simulink model "PmsmFem_testHarness"  (R2024b)
settings: Solver=daessc  StartTime=0.0  StopTime=0.2  RelTol=1e-3  AbsTol=1e-3
libraries: fl_lib x7, nesl_utility x5, ee_lib x4
settings Model: Creator=The MathWorks, Inc.  LastModifiedBy=isaacito
settings SolverCC: AutoScaleAbsTol=off  AlgebraicLoopSolver=TrustRegion
settings DataIOCC: DSMLogging=off
settings DebuggingCC: UnconnectedInputMsg=warning  UnconnectedOutputMsg=warning  UnconnectedLineMsg=warning  ArithmeticOperatorsInVariantConditions=warning
settings ModelReferenceCC: EnableRefExpFcnMdlSchedulingChecks=on
settings SFSimCC: SimUseLocalCustomCode=off  CustomCodeUndefinedFunction=UseInterfaceOnly
settings RTWCC: RTWUseLocalCustomCode=off  GPUComputeCapability=3.5
settings SimscapeCC: SimscapeLogType=all  SimscapeLogSimulationStatistics=on  SimscapeLogName=logsoutssc  SimscapeLogDataHistory=50000

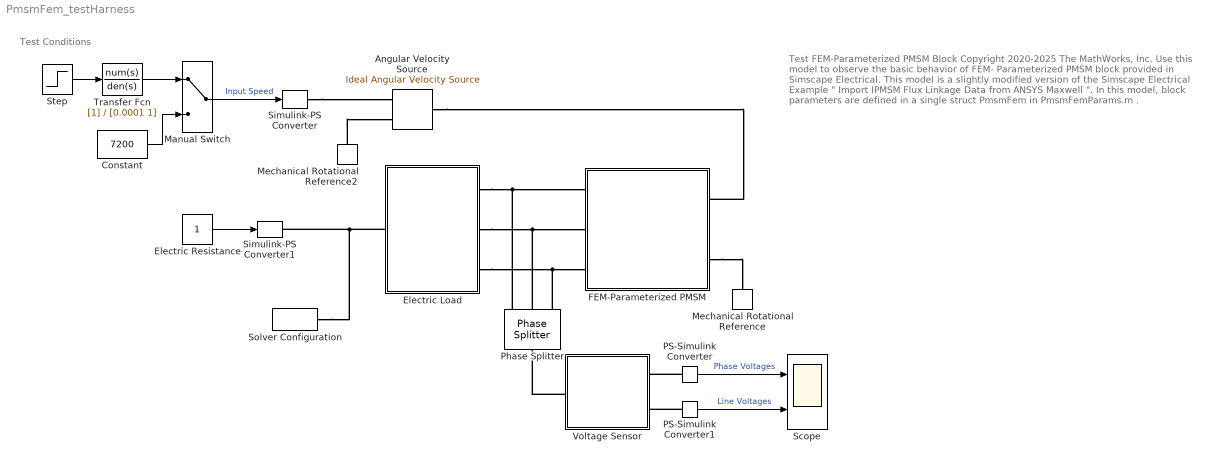
== system PmsmFem_testHarness ==
  note: Test Conditions
  note: Test FEM-Parameterized PMSM Block
      |
      | Copyright 2020-2025 The MathWorks, Inc.
      |
      | Use this model to observe the basic behavior of FEM-
      | Parameterized PMSM block provided in Simscape Electrical.
      | This model is a slightly modified version of the Simscape
      | Electrical Example " Import IPMSM Flux Linkage Data from
      | ANSYS Maxwell ".
      |
      | In this model, block parameters are defined in a single struct
      | PmsmFem in PmsmFemParams.m .
  Angular Velocity Source : fl_lib/Mechanical/Mechanical Sources/Ideal Angular Velocity Source
  Constant : Constant  Value=7200
  Electric Load : Subsystem
  Electric Resistance : Constant
  FEM-Parameterized PMSM : Subsystem  ReferencedSubsystem=PmsmFemRefSub
  Manual Switch : ManualSwitch
  Mechanical Rotational Reference : fl_lib/Mechanical/Rotational Elements/Mechanical Rotational Reference
  Mechanical Rotational Reference2 : fl_lib/Mechanical/Rotational Elements/Mechanical Rotational Reference
  PS-Simulink Converter : nesl_utility/PS-Simulink Converter  PhysicalDomain=network_engine_domain  SubClassName=ps_output  LeftPortType=input  RightPortType=output  PseudoPeriodic=off  Frequencies=[]  VectorFormat=1-D array  Unit=V  AffineConversion=off
  PS-Simulink Converter1 : nesl_utility/PS-Simulink Converter  PhysicalDomain=network_engine_domain  SubClassName=ps_output  LeftPortType=input  RightPortType=output  PseudoPeriodic=off  Frequencies=[]  VectorFormat=1-D array  Unit=V  AffineConversion=off
  Phase Splitter : ee_lib/Connectors & References/Phase Splitter
  Scope : Scope  NumInputPorts=2
  Simulink-PS Converter : nesl_utility/Simulink-PS Converter  PhysicalDomain=network_engine_domain  SubClassName=ps_input  LeftPortType=input  RightPortType=output  PseudoPeriodic=off  Frequencies=[]  NoiseDistribution=none  NoiseParameters=[]  Unit=rpm  AffineConversion=off  FilteringAndDerivatives=filter  SimscapeFilterOrder=1  InputFilterTimeConstant=0.0001  UdotUserProvided=1
  Simulink-PS Converter1 : nesl_utility/Simulink-PS Converter  PhysicalDomain=network_engine_domain  SubClassName=ps_input  LeftPortType=input  RightPortType=output  PseudoPeriodic=off  Frequencies=[]  NoiseDistribution=none  NoiseParameters=[]  Unit=MOhm  AffineConversion=off  FilteringAndDerivatives=provide  SimscapeFilterOrder=1  InputFilterTimeConstant=0.001  UdotUserProvided=0
  Solver Configuration : nesl_utility/Solver Configuration  PhysicalDomain=network_engine_domain  SubClassName=solver  LeftPortType=input  RightPortType=generic  Tones=[]  Harmonics=[]  SimulateNoise=off  Profile=off  UseLocalSampling=off  EnableSwitchedLinearOptims=on  FrequencyDomain=off  UseCCode=off  RelTol=0.001  AbsTol=1e-06  MinStep=1e-09  ToWorkspace=off  RevertToSquareIcSolve=off  NumHomotopyIterations=100  PhasorMode=off  PhasorModeNumHarmonics=1  ConsistencySolver=NEWTON_FTOL  IndexReductionMethod=DerivativeReplacement  DoDC=off  ResidualTolerance=1e-9  ConsistencyTolSource=GLOBAL  ConsistencyAbsTol=0.001  ConsistencyRelTol=0.001  ConsistencyTolFactor=0.001  UseLocalSolver=off  LocalSolverChoice=NE_TRAPEZOIDAL_ADVANCER  ResolveIndetEquations=on  FunctionEvalNumThread=1  LocalSolverSampleTime=0.0001  DoFixedCost=off  MaxNonlinIter=10  MaxModeIter=2  ComputeImpulses=off  ImpulseIterations=2  LinearAlgebra=auto  LinearAlgebraNumThread=0  EquationFormulation=NE_TIME_EF  DelaysMemoryBudget=1024  AutomaticFiltering=on  FilteringTimeConstant=0.001  PartitionStorageMethod=AS_NEEDED  PartitionMemoryBudget=1024  PartitionMethod=FAST  MultibodyUseLocalSolver=off  MultibodyLocalSolverChoice=ODE1  MultibodyLocalSolverSampleTime=0.001
      settings: AttributesFormatString=Local solver %<UseLocalSolver>
  Step : Step  Time=0.1  Before=500  After=1500  SampleTime=0
      settings: AttributesFormatString=|
      | Initial %<Before>
      | Step to %<After>
  Transfer Fcn : TransferFcn  Denominator=[0.0001 1]
  Voltage Sensor : Subsystem
  wires:
  Electric Resistance/1 -> Simulink-PS Converter1/1
  PS-Simulink Converter/1 -> Scope/1  "Phase Voltages"
  PS-Simulink Converter1/1 -> Scope/2  "Line Voltages"
  Manual Switch/1 -> Simulink-PS Converter/1  "Input Speed"
  Transfer Fcn/1 -> Manual Switch/1
  Step/1 -> Transfer Fcn/1
  Constant/1 -> Manual Switch/2
  connections:
  Simulink-PS Converter/RConn1 -- Angular Velocity Source/RConn1
  Mechanical Rotational Reference2/LConn1 -- Angular Velocity Source/RConn2
  Electric Load/LConn1 -- Solver Configuration/RConn1 -- Simulink-PS Converter1/RConn1
  Electric Load/RConn1 -- FEM-Parameterized PMSM/LConn1 -- Phase Splitter/RConn1
  Electric Load/RConn2 -- FEM-Parameterized PMSM/LConn2 -- Phase Splitter/RConn2
  Electric Load/RConn3 -- FEM-Parameterized PMSM/LConn3 -- Phase Splitter/RConn3
  Voltage Sensor/LConn1 -- Phase Splitter/LConn1
  PS-Simulink Converter/LConn1 -- Voltage Sensor/RConn1
  PS-Simulink Converter1/LConn1 -- Voltage Sensor/RConn2
  Angular Velocity Source/LConn1 -- FEM-Parameterized PMSM/RConn1
  FEM-Parameterized PMSM/RConn2 -- Mechanical Rotational Reference/LConn1

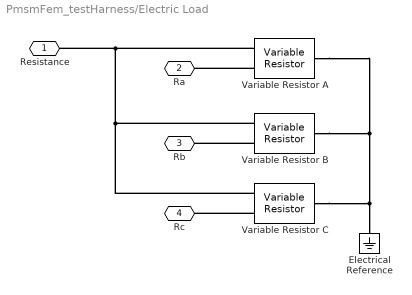
== system PmsmFem_testHarness/Electric Load ==
  Electrical Reference : fl_lib/Electrical/Electrical Elements/Electrical Reference
  Variable Resistor A : fl_lib/Electrical/Electrical Elements/Variable Resistor  Rmin=0 Ohm  thermalEnable=false  thermal_mass=1 J/K  i_specify=off  i_priority=None  i=0 A  i_nominal_specify=off  i_nominal_value=1  i_nominal_unit=A  v_specify=off  v_priority=None  v=0 V  v_nominal_specify=off  v_nominal_value=1  v_nominal_unit=V  T_specify=off  T_priority=None  T=300 K  T_nominal_specify=off  T_nominal_value=1  T_nominal_unit=K
  Variable Resistor B : fl_lib/Electrical/Electrical Elements/Variable Resistor  Rmin=0 Ohm  thermalEnable=false  thermal_mass=1 J/K  i_specify=off  i_priority=None  i=0 A  i_nominal_specify=off  i_nominal_value=1  i_nominal_unit=A  v_specify=off  v_priority=None  v=0 V  v_nominal_specify=off  v_nominal_value=1  v_nominal_unit=V  T_specify=off  T_priority=None  T=300 K  T_nominal_specify=off  T_nominal_value=1  T_nominal_unit=K
  Variable Resistor C : fl_lib/Electrical/Electrical Elements/Variable Resistor  Rmin=0 Ohm  thermalEnable=false  thermal_mass=1 J/K  i_specify=off  i_priority=None  i=0 A  i_nominal_specify=off  i_nominal_value=1  i_nominal_unit=A  v_specify=off  v_priority=None  v=0 V  v_nominal_specify=off  v_nominal_value=1  v_nominal_unit=V  T_specify=off  T_priority=None  T=300 K  T_nominal_specify=off  T_nominal_value=1  T_nominal_unit=K
  Resistance : PMIOPort  Side=Left
  Ra : PMIOPort  Port=2  Side=Right
  Rb : PMIOPort  Port=3  Side=Right
  Rc : PMIOPort  Port=4  Side=Right
  connections:
  Variable Resistor A/LConn1 -- Resistance/RConn1 -- Variable Resistor C/LConn1 -- Variable Resistor B/LConn1
  Variable Resistor A/LConn2 -- Ra/RConn1
  Variable Resistor A/RConn1 -- Variable Resistor C/RConn1 -- Electrical Reference/LConn1 -- Variable Resistor B/RConn1
  Variable Resistor B/LConn2 -- Rb/RConn1
  Variable Resistor C/LConn2 -- Rc/RConn1

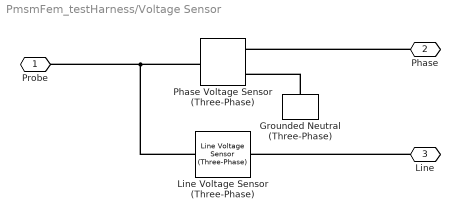
== system PmsmFem_testHarness/Voltage Sensor ==
  Grounded Neutral (Three-Phase) : ee_lib/Connectors & References/Grounded Neutral (Three-Phase)
  Line Voltage Sensor (Three-Phase) : ee_lib/Sensors & Transducers/Line Voltage Sensor (Three-Phase)
  Phase Voltage Sensor (Three-Phase) : ee_lib/Sensors & Transducers/Phase Voltage Sensor (Three-Phase)
  Probe : PMIOPort  Side=Left
  Phase : PMIOPort  Port=2  Side=Right
  Line : PMIOPort  Port=3  Side=Right
  connections:
  Grounded Neutral (Three-Phase)/LConn1 -- Phase Voltage Sensor (Three-Phase)/RConn2
  Phase/RConn1 -- Phase Voltage Sensor (Three-Phase)/RConn1
  Phase Voltage Sensor (Three-Phase)/LConn1 -- Probe/RConn1 -- Line Voltage Sensor (Three-Phase)/LConn1
  Line/RConn1 -- Line Voltage Sensor (Three-Phase)/RConn1
